simulink model "clap_clap_on_off_arduino_nano_R2022a_windows"  (R2022a)
settings: Solver=FixedStepAuto  StartTime=0.0  StopTime=inf  FixedStep=0.005  RelTol=1e-3  EnableMultiTasking=on
libraries: arduinolib x4, simulink_extras x1, eeGeneralControl x1
settings Model: ExtModeTrigDuration=2  Creator=byoun  LastModifiedBy=byoun
settings OptimizationCC: EnhancedBackFolding=on  PassReuseOutputArgsAs=Individual arguments  ZeroExternalMemoryAtStartup=off  ZeroInternalMemoryAtStartup=off  MaxStackSize=64  OptimizeBlockOrder=speed  DifferentSizesBufferReuse=on  OptimizationCustomize=off  EfficientTunableParamExpr=on
settings DebuggingCC: ParameterTunabilityLossMsg=error
settings HardwareCC: ProdBitPerInt=16  ProdBitPerPointer=16  ProdBitPerSizeT=16  ProdBitPerPtrDiffT=16  ProdLargestAtomicFloat=None  ProdWordSize=8  ProdHWDeviceType=Atmel->AVR
settings SFSimCC: MATLABDynamicMemAlloc=off
settings RTWCC: SystemTargetFile=ert.tlc  HardwareBoard=Arduino Nano 3.0  TemplateMakefile=ert_default_tmf  Toolchain=Arduino AVR  BuildConfiguration=Faster Runs
settings CodeAppCC: ForceParamTrailComments=on  IgnoreCustomStorageClasses=off  OperatorAnnotations=on  SimulinkDataObjDesc=on  SFDataObjDesc=on  InsertBlockDesc=on
settings ERTTargetCC: SupportContinuousTime=on  SupportVariableSizeSignals=on  ExtModeTransport=3  ExtModeStaticAlloc=on  ExtModeStaticAllocSize=250  ExtModeMexFile=ext_xcp  ExtModeIntrfLevel=Level2 - Open

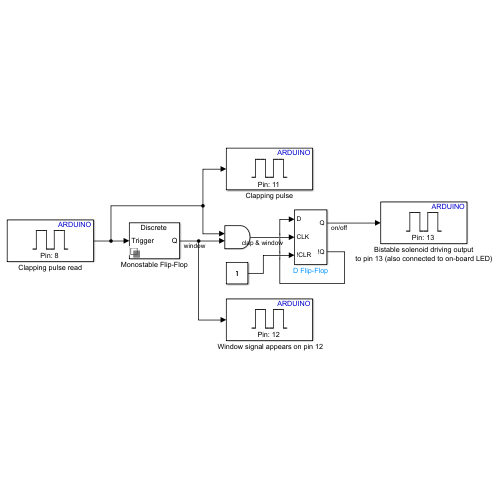
[thumbnail: Simulink's stored preview of the top-level diagram]
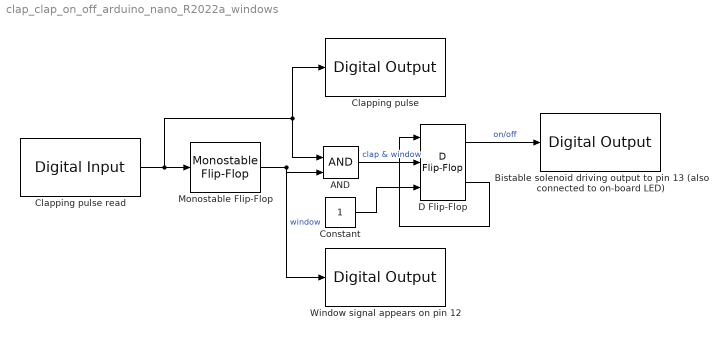
== system clap_clap_on_off_arduino_nano_R2022a_windows ==
  " Window signal appears on pin 12" : arduinolib/Digital Output  pinNumber=12  Direction=output  blockPlatform=arduino
  AND : Logic  IconShape=distinctive  AllPortsSameDT=off  OutDataTypeStr=boolean
  Bistable solenoid driving output to pin 13 (also connected to on-board LED) : arduinolib/Digital Output  pinNumber=13  Direction=output  blockPlatform=arduino
  Clapping pulse : arduinolib/Digital Output  pinNumber=11  Direction=output  blockPlatform=arduino
  Clapping pulse read : arduinolib/Digital Input  pinNumber=8  mode=Default  Direction=input  SampleTime=0.005  blockPlatform=arduino
  Constant : Constant
  D Flip-Flop : simulink_extras/Flip Flops/D Flip-Flop
  Monostable Flip-Flop : eeGeneralControl/Monostable Flip-Flop  VariantControl=Variant1  LabelModeActiveChoice=Discrete  ChangeType=Falling edge  x0=0  Td=0.4  Ts=0.005
      settings: SourceProductBaseCode=PS
  wires:
  Clapping pulse read/1 -> AND/1, Clapping pulse/1, Monostable Flip-Flop/1
  Monostable Flip-Flop/1 -> " Window signal appears on pin 12"/1, AND/2  "window"
  AND/1 -> D Flip-Flop/2  "clap & window"
  D Flip-Flop/2 -> D Flip-Flop/1
  Constant/1 -> D Flip-Flop/3
  D Flip-Flop/1 -> Bistable solenoid driving output to pin 13 (also connected to on-board LED)/1  "on/off"
